simulink model "PhysicsBased_Tutorials"  (R2021a)
settings: Solver=FixedStepAuto  StartTime=0.0  StopTime=50  FixedStep=.0015  RelTol=1e-3
undefined symbols (not defined in the file): Ion, Li
libraries: PB_Library_Master x57, Lib_Solve_SSNRSolverJC_EMTAT x6, Lib_Solve_SSNRSolverJC_TMATS x1, TemperatureBlock x1
(part 2 of 2)

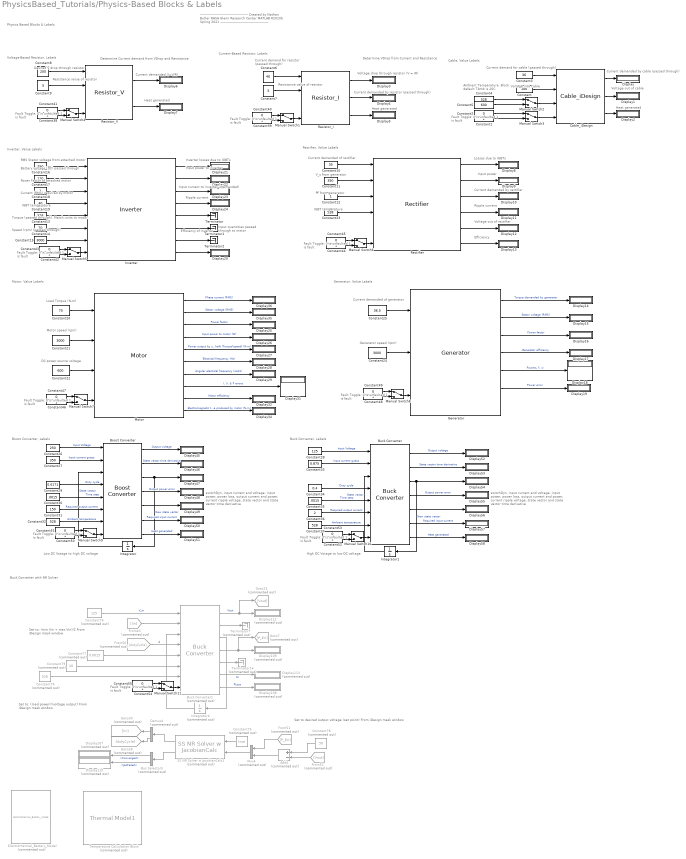
== system PhysicsBased_Tutorials/Physics-Based Blocks & Labels ==
  note: Generator, Value Labels
  note: Current demanded of generator
  note: Rectifier, Value Labels
  note: Current demanded of rectifier
  note: Current demanded by rectifier
  note: Low DC Votage to high DC voltage
  note: switchDyn, input current and voltage, input power, power loss, output current and power, current ripple voltage, state vector and state vector time derivative
  note: Current demanded by cable (passed through)
  note: Heat generated
  note: Voltage out of cable
  note: Voltage into cable
  note: Fault Toggle:
      | 0 is unfaulted
      | 1 is fault
  note: Ambient Temperature.
      | Block default TAmb is 20C
  note: Cable, Value Labels
  note: Current demand for cable (passed through)
  note: Efficiency of inverter
  note: Input quantities passed through to motor
  note: Ripple current
  note: Input current to inverter (Idemanded)
  note: Input power to inverter
  note: Inverter losses due to IGBTs
  note: Speed (rpm) (passed through)
  note: Torque (passed through). Match units to motor.
  note: IGBT temperature
  note: Current (RMS) required by motor
  note: Power Factor of attached motor
  note: Battery voltage (DC) passed through
  note: Resistance value of resistor
  note: Heat generated
  note: Boost Converter, Labels
  note: Current demand for resistor (passed through)
  note: Voltage drop through resistor (V = IR)
  note: Current-Based Resistor, Labels
  note: Determine VDrop from Current and Resistance
  note: Determine Current demand from VDrop and Resistance
  note: Voltage-Based Resistor, Labels
  note: Desired V drop through resistor
  note: Resistance value of resistor
  note: Current demanded (I=V/R)
  note: Heat generated
  note: Current demanded by resistor (passed through)
  note: RMS Stator voltage from attached motor
  note: Inverter, Value Labels
  note: Physics Based Blocks & Labels
  note: Motor speed (rpm)
  note: Motor, Value Labels
  note: Load Torque (N-m)
  note: DC power source voltage
  note: switchDyn, input current and voltage, input power, power loss, output current and power, current ripple voltage, state vector and state vector time derivative
  note: Buck Converter, Labels
  note: High DC Votage to low DC voltage
  note: ------------------------------------------------
      | Created by Nathan Butler
      | NASA Glenn Research Center
      | MATLAB R2020b
      | Spring 2021
      | ------------------------------------------------
  note: Set to desired output voltage (set point)
      | From iDesign mask window
  note: Buck Converter with NR Solver
  note: Set to:
      | (load power)/(voltage output)
      | From iDesign mask window
  note: Set to:
      | (min Vin + max Vin)/2
      | From iDesign mask window
  note: Losses due to IGBTs
  note: Input power
  note: Ripple current
  note: Voltage out of rectifier
  note: Efficiency
  note: V_s from generator
  note: PF from generator
  note: IGBT temperature
  note: Generator speed (rpm)
  note: Fault Toggle:
      | 0 is unfaulted
      | 1 is fault
  note: Fault Toggle:
      | 0 is unfaulted
      | 1 is fault
  note: Fault Toggle:
      | 0 is unfaulted
      | 1 is fault
  note: Fault Toggle:
      | 0 is unfaulted
      | 1 is fault
  note: Fault Toggle:
      | 0 is unfaulted
      | 1 is fault
  note: Fault Toggle:
      | 0 is unfaulted
      | 1 is fault
  note: Fault Toggle:
      | 0 is unfaulted
      | 1 is fault
  note: Fault Toggle:
      | 0 is unfaulted
      | 1 is fault
  note: Fault Toggle:
      | 0 is unfaulted
      | 1 is fault
  Add4 : Sum  Commented=on  Inputs=+-
  Boost Converter : PB_Library_Master/Boost Converter  Pdis_M=1  C_M=1.65e-07  L_M=0.00011412  Ron_M=0.0092  RC_M=0.037475  RL_M=0.03635  QgTotal_M=7.4e-08  Vdiode_M=1.4  TRise_M=7e-09  TFall_M=1e-08  Fsw_M=250000  Vgate_M=3.5  n_MOSFET=1  MassEst_M=37.515  TempIn=Celsius  vOut=540  pow=10000  minV=240  maxV=260  rippleMode=Use defaults (5% of voltage output and 10% of inductor current)  vRip=.05  iRip=.1  freqMode=Use default frequency (250 kHz)  freq=250e3
  Buck Converter : PB_Library_Master/Buck Converter  Pdis_M=1  C_M=0.37515  L_M=4.4e-08  Ron_M=0.0006  RC_M=0.13  RL_M=0.286  QgTotal_M=0.18923  Vgate_M=250000  TRise_M=5e-09  TFall_M=2.3e-08  Fsw_M=2.2e-08  Trr_M=4  n_MOSFET=2.22e-07  MassEst_M=0  TempIn=Celsius  vOut=50  pow=100  minV=123  maxV=127  rippleMode=Use defaults (5% of voltage output and 10% of inductor current)  vRip=.05  iRip=.1  freqMode=Use default frequency (250 kHz)  freq=250e3
  Buck Converter1 : PB_Library_Master/Buck Converter  Commented=on  Pdis_M=1  C_M=4.07e-07  L_M=6e-05  Ron_M=0.0009  RC_M=0.030919  RL_M=0.019013  QgTotal_M=5.8e-08  Vgate_M=1.9  TRise_M=2.2e-08  TFall_M=4.4e-08  Fsw_M=250000  Trr_M=7.7e-08  n_MOSFET=1  MassEst_M=3.7515  TempIn=Celsius  vOut=50  pow=1000  minV=123  maxV=127  rippleMode=Use defaults (5% of voltage output and 10% of inductor current)  vRip=.05  iRip=.1  freqMode=Use default frequency (250 kHz)  freq=250e3
  Bus Selector5 : BusSelector  Commented=on  OutputSignals=Converged,JacFailed
  Cable_iDesign : PB_Library_Master/Cable_iDesign  rad_c_M=0.94407  t_i_M=1.0013  Mass_M=159.0996  R_init=0.006  alpha=0.00393  V_in=120  V_drop=.3  I_out=40  Len=100  FS=1.5  Mat_c=Copper  UResis=0  UDens_C=0  UAlpha=0  Mat_i=PVC  UDens_I=0  UEpsilon=0
  Constant : Constant  Value=100
  Constant{1,12,18,38..39,42,44,46,48,50,52,54} (12 alike) : Constant
  Constant10 : Constant  Value=35
  Constant11 : Constant  Value=350
  Constant{4,13,23,32,37} (5 alike) : Constant  Value=528
  Constant14 : Constant  Value=70
  Constant15 : Constant  Value=3000
  Constant16 : Constant  Value=350
  Constant17 : Constant  Value=120
  Constant19 : Constant  Value=40
  Constant{2,40..41,43,45,47,49,51,53,55} (10 alike) : Constant  Value=0
  Constant20 : Constant  Value=70
  Constant21 : Constant  Value=3000
  Constant22 : Constant  Value=600
  Constant24 : Constant  Value=3000
  Constant25 : Constant  Value=36.5
  Constant26 : Constant  Value=250
  Constant27 : Constant  Value=350
  Constant28 : Constant  Value=125
  Constant29 : Constant  Value=0.6171
  Constant3 : Constant  Value=36
  Constant30 : Constant  Value=.0015
  Constant31 : Constant  Value=150
  Constant33 : Constant  Value=0.875
  Constant34 : Constant  Value=0.4
  Constant35 : Constant  Value=.0015
  Constant36 : Constant  Value=2
  Constant5 : Constant  Value=600
  Constant6 : Constant  Value=40
  Constant7 : Constant  Value=5
  Constant74 : Constant  Commented=on  Value=528
  Constant75 : Constant  Commented=on  Value=true
  Constant76 : Constant  Commented=on  Value=125  VectorParams1D=off  SampleTime=-1
  Constant77 : Constant  Commented=on  Value=0.0015  VectorParams1D=off
  Constant78 : Constant  Commented=on  Value=50
  Constant79 : Constant  Commented=on  Value=20
  Constant8 : Constant  Value=200
  Constant9 : Constant  Value=5
  Demux4 : Demux  Commented=on  Outputs=2
  Display{,1..29,31..32,34..36,45..58} (49 alike) : Display
  Display{107..110,112..113} (6 alike) : Display  Commented=on
  Electrothermal_Battery_Model : PB_Library_Master/Electrothermal_Battery_Model  Commented=on  E0_M=E0_M  Q_M=Q_M  R_M=R_M  K_M=K_M  B_M=B_M  SOC_Init_M=SOC_Init_M  A_M=A_M  battery_type_M=Li-Ion  TempIn=Celsius  BWS=on  thermal=on  nameField=Thermal Model
  From43 : From  Commented=on  GotoTag=Iin
  From50 : From  Commented=on  GotoTag=dutyCycle
  From51 : From  Commented=on  GotoTag=P_Err
  From52 : From  Commented=on  GotoTag=Vout
  Generator : PB_Library_Master/Generator  pp=3  flux_m=0.38515  R_s=0.032  L_s=0.00115  P_Fe_Nom=904.3614  S_nom=4000  T_nom=70  P_out_max=22000  I_max=36.5  P_in_max=30000  T_max=80  MassEst_M=-1080970  Poles_i=6  R_s_i=.032  L_s_i=.00086+0.00029  S_nom_i=4000  T_nom_i=70  P_out_max_i=22000  I_max_i=36.5  P_in_max_i=30000  K_i=121  V_nom_i=368  T_max_i=80  CalculatePFe=Compute iron losses automatically  P_Fe_Nom_i=0  I_nom_i=36.5  PF_nom_i=0.99  P_Fe_Calc_Flag=1
  Goto23 : Goto  Commented=on  GotoTag=Vout
  Goto28 : Goto  Commented=on  GotoTag=dutyCycle
  Goto30 : Goto  Commented=on  GotoTag=Iin
  Goto7 : Goto  Commented=on  GotoTag=P_Err
  Integrator : Integrator
  Integrator1 : Integrator
  Integrator4 : Integrator  Commented=on  InitialCondition=[0;0]
  Inverter : PB_Library_Master/Inverter  T_M=[25 175]  u_D_M=[1.16666666666667 0.999999999999998]  u_ce0_M=[0.971428571428571 0.848275862068965]  R_c_M=[0.0285714285714286 0.0551724137931034]  R_D_M=[0.0238095238095238 0.0294117647058824]  E0_M=[6.00000000000002e-05 6.00000000000002e-05]  E1_M=[5.6e-05 5.6e-05]  f_sw_M=20000  L_s_M=0.1  P_max_I=22000  V_phase_I=600  f_sw_I=0  L_s_I=0.1
  Manual Switch{1..11} (11 alike) : ManualSwitch
  Motor : PB_Library_Master/Motor  pp=2.5  flux_m=0.46219  R_s=0.032  L_s=0.00115  P_Fe_Nom=904.3614  S_nom=3000  T_nom=70  P_out_max=22000  I_max=36.5  P_in_max=30000  T_max=80  MassEst_M=136.5892  Poles_i=5  R_s_i=.032  L_s_i=.00086+0.00029  S_nom_i=3000  T_nom_i=70  P_out_max_i=22000  I_max_i=36.5  P_in_max_i=30000  K_i=121  V_nom_i=368  T_max_i=80  CalculatePFe=Compute iron losses automatically  P_Fe_Nom_i=0  I_nom_i=36.5  PF_nom_i=0.99  P_Fe_Calc_Flag=1
  Mux4 : Mux  Commented=on  Inputs=2
  Rectifier : PB_Library_Master/Rectifier  T_M=[25 175]  u_D_M=[1.16666666666667 0.999999999999998]  u_ce0_M=[0.971428571428571 0.848275862068965]  R_c_M=[0.0285714285714286 0.0551724137931034]  R_D_M=[0.0238095238095238 0.0294117647058824]  E0_M=[6.00000000000002e-05 6.00000000000002e-05]  E1_M=[5.6e-05 5.6e-05]  f_sw_M=20000  L_s_M=0.1  P_max_I=22000  V_phase_I=600  f_sw_I=0  L_s_I=0.1
  Resistor_I : PB_Library_Master/Resistor_I  TempIn=Celsius
  Resistor_V : PB_Library_Master/Resistor_V  TempIn=Celsius
  SS NR Solver w JacobianCalc1 : Lib_Solve_SSNRSolverJC_TMATS/SS NR Solver w JacobianCalc  Commented=on  SJac_Per_M=[.01, .001; -.01, -.001]  SNR_IC_M=[5;0.5]  SNR_DX_M=1  SNR_Mx_M=[100000;0.99999]  SNR_Mn_M=[0.00001;0.00001]  SJacobianAttempts_M=200  Cond_Limits_M=0.0001
  Temperature Calculation Block : TemperatureBlock/Thermal Model1  Commented=on  Tj_0_M=25  Ts_0_M=25  Cj_M=Cj  Rj_M=Rj  Ru_M=Ru  Cs_M=Cs
  Terminator : Terminator
  Terminator1 : Terminator
  Terminator14 : Terminator  Commented=on
  Terminator2 : Terminator
  Terminator7 : Terminator  Commented=on
  wires:
  Constant17/1 -> Inverter/2
  Constant2/1 -> Manual Switch3/1
  Manual Switch2/1 -> Cable_iDesign/3
  Resistor_V/2 -> Display7/1
  Resistor_I/2 -> Display4/1
  Cable_iDesign/1 -> Display/1
  Constant15/1 -> Inverter/7
  Resistor_V/1 -> Display6/1
  Inverter/7 -> Terminator2/1
  Cable_iDesign/2 -> Display1/1
  Constant7/1 -> Resistor_I/2
  Constant14/1 -> Inverter/6
  Constant3/1 -> Cable_iDesign/1
  Constant5/1 -> Manual Switch2/2
  Resistor_I/1 -> Display3/1
  Resistor_I/3 -> Display5/1
  Manual Switch3/1 -> Cable_iDesign/4
  Constant1/1 -> Manual Switch3/2
  Constant19/1 -> Inverter/4
  Cable_iDesign/3 -> Display2/1
  Inverter/4 -> Display24/1
  Constant13/1 -> Inverter/5
  Constant4/1 -> Manual Switch2/1
  Constant9/1 -> Resistor_V/2
  Inverter/1 -> Display21/1
  Constant/1 -> Cable_iDesign/2
  Inverter/3 -> Display23/1
  Constant8/1 -> Resistor_V/1
  Constant6/1 -> Resistor_I/1
  Inverter/8 -> Display20/1
  Inverter/2 -> Display22/1
  Constant16/1 -> Inverter/1
  Constant18/1 -> Inverter/3
  Inverter/6 -> Terminator1/1
  Inverter/5 -> Terminator/1
  Motor/1 -> Display36/1  "Phase current (RMS)"
  Constant20/1 -> Motor/1
  Motor/5 -> Display27/1  "Power output by shaft (Torque*speed) (N-m)"
  Motor/2 -> Display35/1  "Stator voltage (RMS)"
  Motor/4 -> Display26/1  "Input power to motor (W)"
  Motor/7 -> Display29/1  "Angular electrical frequency (rad/s)"
  Motor/3 -> Display25/1  "Power factor"
  Constant21/1 -> Motor/2
  Motor/10 -> Display34/1  "Electromagnetic torque produced by motor (N-m)"
  Motor/6 -> Display28/1  "Electrical frequency (Hz)"
  Constant22/1 -> Motor/3
  Motor/9 -> Display32/1  "Motor efficiency"
  Motor/8 -> Display31/1  "I, V, & P errors"
  Constant26/1 -> Boost Converter/1  "Input Voltage"
  Constant27/1 -> Boost Converter/2  "Input current guess"
  Integrator/1 -> Boost Converter/3  "State vector"
  Constant29/1 -> Boost Converter/4  "Duty cycle"
  Constant30/1 -> Boost Converter/5  "Time step"
  Constant31/1 -> Boost Converter/6  "Required output current"
  Constant32/1 -> Boost Converter/7  "Ambient temperature"
  Boost Converter/1 -> Display45/1  "Output voltage"
  Boost Converter/2 -> Display46/1  "State vector time derivative"
  Boost Converter/3 -> Display47/1, Integrator/1  "New state vector"
  Boost Converter/4 -> Display48/1  "Output power error"
  Boost Converter/5 -> Display49/1
  Boost Converter/6 -> Display50/1  "Required input current"
  Boost Converter/7 -> Display51/1  "Heat generated"
  Buck Converter/7 -> Display58/1  "Heat generated"
  Buck Converter/1 -> Display52/1  "Output voltage"
  Buck Converter/6 -> Display57/1  "Required input current"
  Constant37/1 -> Buck Converter/7  "Ambient temperature"
  Constant35/1 -> Buck Converter/5  "Time step"
  Buck Converter/4 -> Display55/1  "Output power error"
  Constant28/1 -> Buck Converter/1  "Input Voltage"
  Integrator1/1 -> Buck Converter/3  "State vector"
  Buck Converter/5 -> Display56/1
  Buck Converter/2 -> Display53/1  "State vector time derivative"
  Constant33/1 -> Buck Converter/2  "Input current guess"
  Constant34/1 -> Buck Converter/4  "Duty cycle"
  Constant36/1 -> Buck Converter/6  "Required output current"
  Buck Converter/3 -> Display54/1, Integrator1/1  "New state vector"
  Constant75/1 -> SS NR Solver w JacobianCalc1/1
  Add4/1 -> Mux4/2
  Constant78/1 -> Add4/1
  SS NR Solver w JacobianCalc1/1 -> Demux4/1
  From43/1 -> Buck Converter1/2
  Buck Converter1/3 -> Integrator4/1
  Bus Selector5/1 -> Display107/1  "<Converged>"
  Demux4/2 -> Goto28/1
  From50/1 -> Buck Converter1/4  "d"
  Buck Converter1/2 -> Terminator7/1
  Constant79/1 -> Buck Converter1/6
  Buck Converter1/1 -> Goto23/1, Display112/1  "Vout"
  From52/1 -> Add4/2
  Constant76/1 -> Buck Converter1/1  "V_in"
  From51/1 -> Mux4/1
  Buck Converter1/6 -> Display113/1  "Iin"
  Buck Converter1/5 -> Terminator14/1
  Demux4/1 -> Goto30/1
  SS NR Solver w JacobianCalc1/2 -> Bus Selector5/1
  Buck Converter1/4 -> Goto7/1, Display109/1
  Integrator4/1 -> Buck Converter1/3
  Mux4/1 -> SS NR Solver w JacobianCalc1/2
  Constant77/1 -> Buck Converter1/5
  Constant74/1 -> Buck Converter1/7
  Buck Converter1/7 -> Display108/1  "PLoss"
  Bus Selector5/2 -> Display110/1  "<JacFailed>"
  Rectifier/1 -> Display8/1
  Rectifier/2 -> Display9/1
  Rectifier/3 -> Display10/1
  Rectifier/4 -> Display11/1
  Rectifier/6 -> Display13/1
  Rectifier/5 -> Display12/1
  Constant10/1 -> Rectifier/1
  Constant11/1 -> Rectifier/2
  Constant12/1 -> Rectifier/3
  Constant23/1 -> Rectifier/4
  Constant24/1 -> Generator/2
  Constant25/1 -> Generator/1
  Generator/1 -> Display14/1  "Torque demanded by generator"
  Generator/2 -> Display15/1  "Stator voltage (RMS)"
  Generator/3 -> Display16/1  "Power factor"
  Generator/4 -> Display17/1  "Generator efficiency"
  Generator/5 -> Display18/1  "Powers, f, w"
  Generator/6 -> Display19/1  "Power error"
  Constant39/1 -> Manual Switch1/2
  Constant40/1 -> Manual Switch1/1
  Manual Switch1/1 -> Resistor_I/4
  Constant38/1 -> Manual Switch4/2
  Manual Switch4/1 -> Resistor_V/4
  Constant41/1 -> Manual Switch4/1
  Constant42/1 -> Manual Switch5/2
  Manual Switch5/1 -> Inverter/8
  Constant43/1 -> Manual Switch5/1
  Constant44/1 -> Manual Switch6/2
  Manual Switch6/1 -> Rectifier/6
  Constant45/1 -> Manual Switch6/1
  Constant46/1 -> Manual Switch7/2
  Manual Switch7/1 -> Motor/4
  Constant47/1 -> Manual Switch7/1
  Constant48/1 -> Manual Switch8/2
  Manual Switch8/1 -> Generator/3
  Constant49/1 -> Manual Switch8/1
  Constant50/1 -> Manual Switch9/2
  Manual Switch9/1 -> Boost Converter/8
  Constant51/1 -> Manual Switch9/1
  Constant52/1 -> Manual Switch10/2
  Manual Switch10/1 -> Buck Converter/8
  Constant53/1 -> Manual Switch10/1
  Constant54/1 -> Manual Switch11/2
  Manual Switch11/1 -> Buck Converter1/8
  Constant55/1 -> Manual Switch11/1

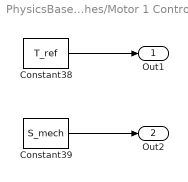
== system PhysicsBased_Tutorials/Example 1: Multiple Motor Branches/Motor 1 Control ==
  Constant38 : Constant  Value=T_ref
  Constant39 : Constant  Value=S_mech
  Out1 : Outport
  Out2 : Outport  Port=2
  wires:
  Constant38/1 -> Out1/1
  Constant39/1 -> Out2/1

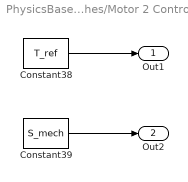
== system PhysicsBased_Tutorials/Example 1: Multiple Motor Branches/Motor 2 Control ==
  Constant38 : Constant  Value=T_ref
  Constant39 : Constant  Value=S_mech
  Out1 : Outport
  Out2 : Outport  Port=2
  wires:
  Constant39/1 -> Out2/1
  Constant38/1 -> Out1/1

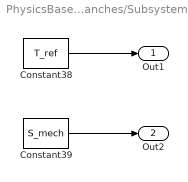
== system PhysicsBased_Tutorials/Example 1: Multiple Motor Branches/Subsystem5 ==
  Constant38 : Constant  Value=T_ref
  Constant39 : Constant  Value=S_mech
  Out1 : Outport
  Out2 : Outport  Port=2
  wires:
  Constant38/1 -> Out1/1
  Constant39/1 -> Out2/1

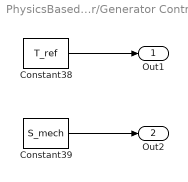
== system PhysicsBased_Tutorials/Example 2: Generator & Rectifier/Generator Control ==
  Constant38 : Constant  Value=T_ref
  Constant39 : Constant  Value=S_mech
  Out1 : Outport
  Out2 : Outport  Port=2
  wires:
  Constant38/1 -> Out1/1
  Constant39/1 -> Out2/1

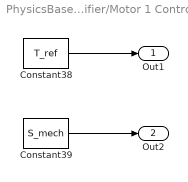
== system PhysicsBased_Tutorials/Example 2: Generator & Rectifier/Motor 1 Control ==
  Constant38 : Constant  Value=T_ref
  Constant39 : Constant  Value=S_mech
  Out1 : Outport
  Out2 : Outport  Port=2
  wires:
  Constant38/1 -> Out1/1
  Constant39/1 -> Out2/1
